simulink model "RC_Circuit"  (R2020a)
settings: Solver=VariableStepAuto  StartTime=0.0  StopTime=10  RelTol=1e-3
settings Model: Creator=DELL  LastModifiedBy=DELL

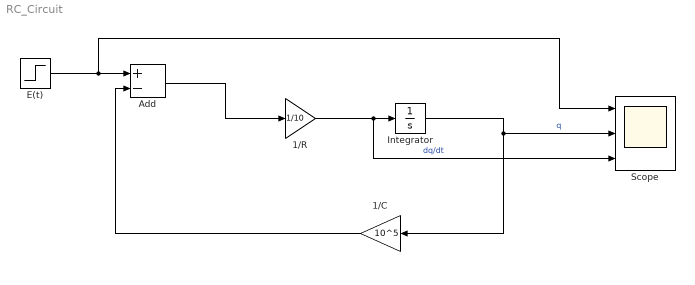
== system RC_Circuit ==
  1/C : Gain  Gain=10^5
  1/R : Gain  Gain=1/10
  Add : Sum  Inputs=+-
  E(t) : Step  SampleTime=0
  Integrator : Integrator
  Scope : Scope  NumInputPorts=3
  wires:
  Add/1 -> 1/R/1
  1/R/1 -> Scope/3, Integrator/1  "dq/dt"
  Integrator/1 -> 1/C/1, Scope/2  "q"
  1/C/1 -> Add/2
  E(t)/1 -> Scope/1, Add/1
